simulink model "simulator"  (R2022b)
settings: Solver=FixedStepAuto  StartTime=0.0  StopTime=1800  FixedStep=1/7000  RelTol=1e-7
undefined symbols (not defined in the file): simdb
libraries: sim_lib x40, simulink_extras x15, matrix_library x9, simulink x1
(part 2 of 3)

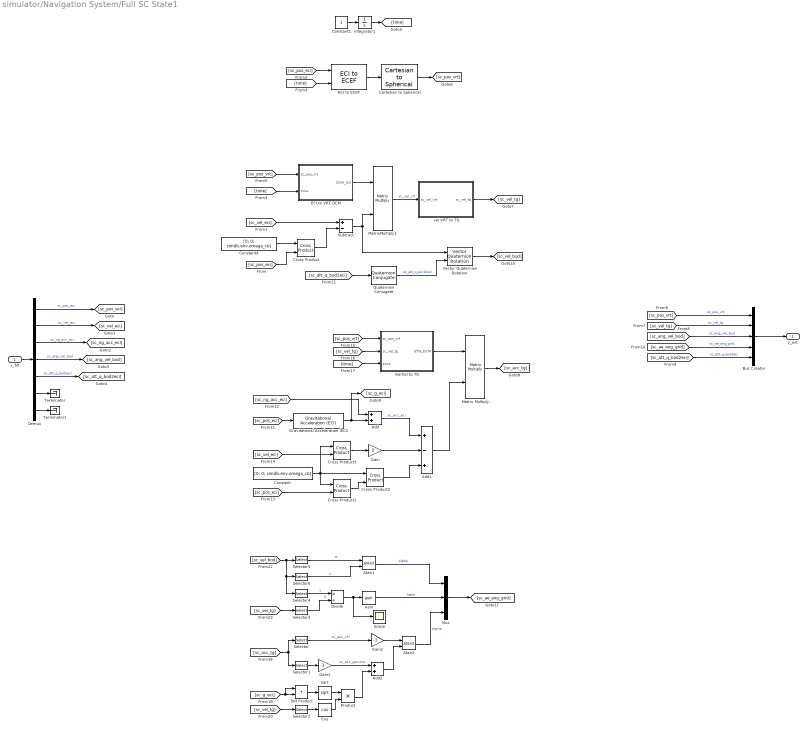
== system simulator/Navigation System/Full SC State1 ==
  x_filt : Inport
  Add : Sum
  Add1 : Sum  Inputs=+-+
  Add2 : Sum
  Asin : Trigonometry  Operator=asin
  Atan1 : Trigonometry  Operator=atan2
  Atan2 : Trigonometry  Operator=atan2
  Bus Creator : BusCreator  Inputs=5
  Cartesian to Spherical : sim_lib/Cartesian to Spherical  SystemSampleTime=-1  VariantActivationTime=update diagram  Latency=0  AutoFrameSizeCalculation=off
  Constant : Constant  Value=[0; 0; simdb.env.omega_cb]
  Constant1 : Constant
  Constant4 : Constant  Value=[0; 0; simdb.env.omega_cb]
  Cos : Trigonometry  Operator=cos
  Cross Product{,1..3} (4 alike) : matrix_library/Cross Product
  Demux : Demux  Outputs=7
  Divide : Product  Inputs=*/
  Dot Product : DotProduct  OutDataTypeStr=Inherit: Inherit via internal rule
  ECI to ECEF : sim_lib/ECI to ECEF  omega_cb=0
  ECI to VRT DCM : Subsystem
  Gain : Gain  Gain=2
  Gain1 : Gain  Gain=-1
  Gain2 : Gain  Gain=-1
  Gravitational Acceleration (ECI) : sim_lib/Gravitational Acceleration (ECI)  mu=simdb.env.mu
  Inertial to TG : Subsystem
  Integrator1 : Integrator
  Matrix Multiply : Product  Multiplication=Matrix(*)
  MatrixMultiply1 : Product  Multiplication=Matrix(*)
  Mux : Mux  Inputs=3
  Product : Product
  Quaternion Conjugate : sim_lib/Quaternion Conjugate  SystemSampleTime=-1  VariantActivationTime=update diagram  Latency=0  AutoFrameSizeCalculation=off
  Scope : Scope
  Selector : Selector  InputPortWidth=3  IndexOptions=Index vector (dialog)  Indices=[2]  OutputSizes=1
  Selector1 : Selector  InputPortWidth=3  IndexOptions=Index vector (dialog)  Indices=[3]  OutputSizes=1
  Selector2 : Selector  InputPortWidth=3  IndexOptions=Index vector (dialog)  Indices=[2]  OutputSizes=1
  Selector3 : Selector  InputPortWidth=3  IndexOptions=Index vector (dialog)  Indices=[1]  OutputSizes=1
  Selector4 : Selector  InputPortWidth=3  IndexOptions=Index vector (dialog)  Indices=[2]  OutputSizes=1
  Selector5 : Selector  InputPortWidth=3  IndexOptions=Index vector (dialog)  Indices=[3]  OutputSizes=1
  Selector6 : Selector  InputPortWidth=3  IndexOptions=Index vector (dialog)  Indices=[1]  OutputSizes=1
  Sqrt : Sqrt
  Subtract : Sum  Inputs=+-
  Terminator : Terminator
  Terminator1 : Terminator
  Vector Quaternion Rotation : sim_lib/Vector Quaternion Rotation  SystemSampleTime=-1  VariantActivationTime=update diagram  Latency=0  AutoFrameSizeCalculation=off
  vel VRT to TG : Subsystem
  y_est : Outport
  wires:
  x_filt/1 -> Demux/1
  Demux/2 -> [sc_vel_eci]  "sc_vel_eci"
  Demux/4 -> [sc_ang_vel_bod]  "sc_ang_vel_bod"
  Demux/5 -> [sc_att_q_bod2eci]  "sc_att_q_bod2eci"
  Demux/6 -> Terminator/1
  Demux/7 -> Terminator1/1
  Bus Creator/1 -> y_est/1
  Constant4/1 -> Cross Product/1
  Cross Product/1 -> Subtract/2
  Demux/1 -> [sc_pos_eci]  "sc_pos_eci"
  Demux/3 -> [sc_ng_acc_eci]  "sc_ng_acc_eci"
  [sc_pos_eci] -> Cross Product/2
  [sc_vel_eci] -> Subtract/1
  Subtract/1 -> MatrixMultiply1/2, Vector Quaternion Rotation/1
  ECI to VRT DCM/1(DCM_I2V) -> MatrixMultiply1/1
  Constant1/1 -> Integrator1/1
  Integrator1/1 -> [time]
  [time] -> ECI to VRT DCM/2(time)
  [sc_pos_eci] -> ECI to ECEF/1
  [time] -> ECI to ECEF/2
  ECI to ECEF/1 -> Cartesian to Spherical/1
  Cartesian to Spherical/1 -> [sc_pos_vrt]
  [sc_pos_vrt] -> ECI to VRT DCM/1(sc_pos_vrt)
  MatrixMultiply1/1 -> vel VRT to TG/1(sc_vel_vrt)  "sc_vel_vrt"
  vel VRT to TG/1(sc_vel_tg) -> [sc_vel_tg]
  [sc_pos_vrt] -> Bus Creator/1  "sc_pos_vrt"
  [sc_vel_tg] -> Bus Creator/2  "sc_vel_tg"
  [sc_ang_vel_bod] -> Bus Creator/3  "sc_ang_vel_bod"
  [sc_att_q_bod2eci] -> Bus Creator/5  "sc_att_q_bod2eci"
  [sc_ae_ang_gnd] -> Bus Creator/4  "sc_ae_ang_gnd"
  [sc_pos_eci] -> Gravitational Acceleration (ECI)/1
  Gravitational Acceleration (ECI)/1 -> Add/2, [sc_g_eci]
  [sc_ng_acc_eci] -> Add/1
  Add/1 -> Add1/1  "sc_acc_eci"
  [sc_pos_eci] -> Cross Product1/2
  Constant/1 -> Cross Product3/1, Cross Product2/1, Cross Product1/1
  Cross Product1/1 -> Cross Product2/2
  [sc_vel_eci] -> Cross Product3/2
  Cross Product3/1 -> Gain/1
  Gain/1 -> Add1/2
  Cross Product2/1 -> Add1/3
  Add1/1 -> Matrix Multiply/2
  [sc_pos_vrt] -> Inertial to TG/1(sc_pos_vrt)
  [sc_vel_tg] -> Inertial to TG/2(sc_vel_tg)
  [time] -> Inertial to TG/3(time)
  Inertial to TG/1(I2TG_DCM) -> Matrix Multiply/1
  Matrix Multiply/1 -> [sc_acc_tg]
  [sc_acc_tg] -> Selector/1, Selector1/1
  Selector/1 -> Gain2/1  "sc_acc_chi"
  Selector1/1 -> Gain1/1
  Gain1/1 -> Add2/1  "sc_acc_gamma"
  [sc_g_eci] -> Dot Product/1, Dot Product/2
  Dot Product/1 -> Sqrt/1
  [sc_vel_tg] -> Selector2/1
  Selector2/1 -> Cos/1
  Sqrt/1 -> Product/1
  Cos/1 -> Product/2
  Product/1 -> Add2/2
  Gain2/1 -> Atan2/1
  Add2/1 -> Atan2/2
  [sc_att_q_bod2eci] -> Quaternion Conjugate/1
  Quaternion Conjugate/1 -> Vector Quaternion Rotation/2  "sc_att_q_eci2bod"
  Vector Quaternion Rotation/1 -> [sc_vel_bod]
  [sc_vel_tg] -> Selector3/1
  [sc_vel_bod] -> Selector4/1, Selector6/1, Selector5/1
  Selector5/1 -> Atan1/1  "w"
  Selector6/1 -> Atan1/2  "u"
  Divide/1 -> Scope/1, Asin/1
  Selector4/1 -> Divide/1  "v"
  Selector3/1 -> Divide/2  "V"
  Atan1/1 -> Mux/1  "alpha"
  Asin/1 -> Mux/2  "beta"
  Atan2/1 -> Mux/3  "sigma"
  Mux/1 -> [sc_ae_ang_gnd]

== system simulator/Navigation System/IMU ==
  Bus Element In : Inport  PortName=dke_out  Element=sc_ng_acc_bod
  Bus Element In1 : Inport  PortName=dke_out  Element=sc_ang_vel_bod
  Accelerometer : Subsystem
  Gyroscope : Subsystem
  Terminator1 : Terminator
  Terminator2 : Terminator
  sen_acc_out : Outport
  sen_gyr_out : Outport  Port=2
  wires:
  Gyroscope/1(sen_gyr_out) -> sen_gyr_out/1
  Accelerometer/1(sen_acc_out) -> sen_acc_out/1
  Bus Element In/1 -> Accelerometer/1(sc_ng_acc_bod)
  Bus Element In1/1 -> Gyroscope/1(sc_ang_vel_bod)
  Gyroscope/2(sen_gyr_rawdata) -> Terminator2/1
  Accelerometer/2(sen_acc_rawdata) -> Terminator1/1

== system simulator/Plant/Aero-Surfaces Model ==
  delta_ae_cmd : Inport
  delta_ae : Outport
  wires:
  delta_ae_cmd/1 -> delta_ae/1

== system simulator/Plant/Forces & Moments ==
  state : Inport
  T : Inport  Port=2
  delta_ae : Inport  Port=3
  Aerodynamics : Subsystem
  Gravitational Force : Subsystem
  Height : sim_lib/Height  Rp=simdb.env.Rp
  RCS : Subsystem
  Selector : Selector  InputPortWidth=16  IndexOptions=Index vector (dialog)  Indices=[4]  OutputSizes=1
  Selector1 : Selector  InputPortWidth=16  IndexOptions=Index vector (dialog)  Indices=[1]  OutputSizes=1
  Selector2 : Selector  InputPortWidth=16  IndexOptions=Index vector (dialog)  Indices=[10]  OutputSizes=1
  Selector3 : Selector  InputPortWidth=16  IndexOptions=Index vector (dialog)  Indices=[11]  OutputSizes=1
  Selector4 : Selector  InputPortWidth=16  IndexOptions=Index vector (dialog)  Indices=[5]  OutputSizes=1
  Selector5 : Selector  InputPortWidth=16  IndexOptions=Index vector (dialog)  Indices=[12]  OutputSizes=1
  Bus Element Out : Outport  PortName=dyn_out  Element=sc_for_rcs_traj
  Bus Element Out1 : Outport  PortName=dyn_out  Element=sc_for_rcs_bod
  Bus Element Out2 : Outport  PortName=dyn_out  Element=sc_tor_rcs_bod
  Bus Element Out3 : Outport  PortName=dyn_out  Element=sc_for_g_traj
  Bus Element Out4 : Outport  PortName=dyn_out  Element=sc_for_ae_traj
  Bus Element Out5 : Outport  PortName=dyn_out  Element=sc_for_ae_bod
  Bus Element Out6 : Outport  PortName=dyn_out  Element=sc_tor_ae_bod
  wires:
  T/1 -> RCS/1(T)
  delta_ae/1 -> Aerodynamics/6(delta_ae)
  RCS/1(sc_for_rcs_traj) -> Bus Element Out/1
  RCS/3(sc_tor_rcs_bod) -> Bus Element Out2/1
  Gravitational Force/1(sc_for_g_traj) -> Bus Element Out3/1
  Selector1/1 -> Gravitational Force/1(R), Height/1  "R"
  Selector3/1 -> Aerodynamics/4(AoS)
  Selector/1 -> Aerodynamics/2(V)
  state/1 -> Selector5/1, Selector3/1, Selector2/1, Selector/1, Selector4/1, Selector1/1
  Selector4/1 -> Gravitational Force/2(gamma)
  Aerodynamics/3(sc_tor_ae_bod) -> Bus Element Out6/1
  Aerodynamics/1(sc_for_ae_traj) -> Bus Element Out4/1
  Height/1 -> Aerodynamics/1(h)
  RCS/2(sc_for_rcs_bod) -> Bus Element Out1/1
  Aerodynamics/2(sc_for_ae_bod) -> Bus Element Out5/1
  Selector2/1 -> Aerodynamics/3(AoA)
  Selector5/1 -> Aerodynamics/5(sigma)

== system simulator/Plant/Non-grav acceleration (bod) ==
  sc_pos_vrt : Inport
  sc_vel_tg : Inport  Port=2
  sc_att_q_bod2eci : Inport  Port=3
  dyn_out : Inport  Port=4
  Add : Sum
  Add1 : Sum
  Add2 : Sum
  Bus Selector2 : BusSelector  OutputSignals=sc_for_rcs_bod,sc_for_ae_bod
  Constant : Constant
  Cross Product : matrix_library/Cross Product
  Cross Product1 : matrix_library/Cross Product
  Cross Product2 : matrix_library/Cross Product
  Divide1 : Product  Inputs=*/
  ECEF to ECI : sim_lib/ECEF to ECI  omega_cb=0
  Gain : Gain  Gain=-1
  Gain1 : Gain  Gain=2
  Integrator : Integrator
  MatrixMultiply : Product  Multiplication=Matrix(*)
  Quaternion Conjugate : sim_lib/Quaternion Conjugate  SystemSampleTime=-1  VariantActivationTime=update diagram  Latency=0  AutoFrameSizeCalculation=off
  SPH 2 CART : sim_lib/Spherical to Cartesian  SystemSampleTime=-1  VariantActivationTime=update diagram  Latency=0  AutoFrameSizeCalculation=off
  VRT to ECI DCM : Subsystem
  Vector Quaternion Rotation : sim_lib/Vector Quaternion Rotation  SystemSampleTime=-1  VariantActivationTime=update diagram  Latency=0  AutoFrameSizeCalculation=off
  omega_cb_vec : Constant  Value=[0; 0; simdb.env.omega_cb]
  sc mass : Constant  Value=simdb.sc.m
  vel TG to VRT : Subsystem
  sc_ng_acc_bod : Outport
  wires:
  Constant/1 -> Integrator/1
  sc_pos_vrt/1 -> VRT to ECI DCM/1(sc_pos_vrt), SPH 2 CART/1
  sc_vel_tg/1 -> vel TG to VRT/1(sc_vel_tg)
  Integrator/1 -> ECEF to ECI/2, VRT to ECI DCM/2(time)
  VRT to ECI DCM/1(DCM_V2I) -> MatrixMultiply/1
  vel TG to VRT/1(sc_vel_vrt) -> MatrixMultiply/2
  MatrixMultiply/1 -> Cross Product2/2  "sc_vel_eci"
  SPH 2 CART/1 -> ECEF to ECI/1
  ECEF to ECI/1 -> Cross Product/2  "sc_pos_eci"
  omega_cb_vec/1 -> Cross Product1/1, Cross Product/1, Cross Product2/1
  Cross Product/1 -> Cross Product1/2
  Cross Product1/1 -> Gain/1
  Cross Product2/1 -> Gain1/1
  sc_att_q_bod2eci/1 -> Quaternion Conjugate/1
  Gain/1 -> Add1/1
  Gain1/1 -> Add1/2
  Add1/1 -> Vector Quaternion Rotation/1
  Quaternion Conjugate/1 -> Vector Quaternion Rotation/2
  dyn_out/1 -> Bus Selector2/1
  Bus Selector2/2 -> Add2/2  "<sc_for_ae_bod>"
  Add2/1 -> Divide1/1
  Bus Selector2/1 -> Add2/1  "<sc_for_rcs_bod>"
  sc mass/1 -> Divide1/2
  Vector Quaternion Rotation/1 -> Add/2
  Divide1/1 -> Add/1
  Add/1 -> sc_ng_acc_bod/1

== system simulator/Plant/Thrusters Model ==
  T_cmd : Inport
  T : Outport
  wires:
  T_cmd/1 -> T/1

== system simulator/Guidance System/Reference Trajectory/Ref Trajectory ==
  t : Inport
  Mux : Mux  Inputs=6
  Ref State (R) : Lookup_n-D  NumberOfTableDimensions=1  BreakpointsForDimension1=gui.t_gui  BreakpointsForDimension2=[1:3]  Table=gui.y_gui(1,:)  RemoveProtectionInput=on  InternalRulePriority=Speed  RndMeth=Simplest
  Ref State (V) : Lookup_n-D  NumberOfTableDimensions=1  BreakpointsForDimension1=gui.t_gui  BreakpointsForDimension2=[1:3]  Table=gui.y_gui(4,:)  RemoveProtectionInput=on  InternalRulePriority=Speed  RndMeth=Simplest
  Ref State (chi) : Lookup_n-D  NumberOfTableDimensions=1  BreakpointsForDimension1=gui.t_gui  BreakpointsForDimension2=[1:3]  Table=gui.y_gui(6,:)  RemoveProtectionInput=on  InternalRulePriority=Speed  RndMeth=Simplest
  Ref State (delta) : Lookup_n-D  NumberOfTableDimensions=1  BreakpointsForDimension1=gui.t_gui  BreakpointsForDimension2=[1:3]  Table=gui.y_gui(3,:)  RemoveProtectionInput=on  InternalRulePriority=Speed  RndMeth=Simplest
  Ref State (gamma) : Lookup_n-D  NumberOfTableDimensions=1  BreakpointsForDimension1=gui.t_gui  BreakpointsForDimension2=[1:3]  Table=gui.y_gui(5,:)  RemoveProtectionInput=on  InternalRulePriority=Speed  RndMeth=Simplest
  Ref State (tau) : Lookup_n-D  NumberOfTableDimensions=1  BreakpointsForDimension1=gui.t_gui  BreakpointsForDimension2=[1:3]  Table=gui.y_gui(2,:)  RemoveProtectionInput=on  InternalRulePriority=Speed  RndMeth=Simplest
  y_ref : Outport
  wires:
  t/1 -> Ref State (R)/1, Ref State (tau)/1, Ref State (delta)/1, Ref State (chi)/1, Ref State (gamma)/1, Ref State (V)/1
  Ref State (R)/1 -> Mux/1
  Ref State (chi)/1 -> Mux/6
  Ref State (tau)/1 -> Mux/2
  Ref State (delta)/1 -> Mux/3
  Ref State (V)/1 -> Mux/4
  Ref State (gamma)/1 -> Mux/5
  Mux/1 -> y_ref/1

== system simulator/Navigation System/Extended Kalman Filter/Covariance Matrix Estimation ==
  F : Inport
  P_prev : Inport  Port=2
  Add : Sum  Inputs=+++
  Matrix Multiply : Product  Multiplication=Matrix(*)
  Matrix Multiply1 : Product  Multiplication=Matrix(*)
  Q matrix : Constant  Value=simdb.nav.Q
  Transpose : Math  Operator=transpose
  P_est : Outport
  wires:
  F/1 -> Transpose/1, Matrix Multiply/1
  Matrix Multiply1/1 -> Add/1
  Matrix Multiply/1 -> Add/2
  P_prev/1 -> Matrix Multiply/2, Matrix Multiply1/1
  Q matrix/1 -> Add/3
  Add/1 -> P_est/1
  Transpose/1 -> Matrix Multiply1/2

== system simulator/Navigation System/Extended Kalman Filter/Covariance Matrix Update ==
  K : Inport
  H : Inport  Port=2
  P_est : Inport  Port=3
  Identity : Constant  Value=eye(22)
  Matrix Multiply : Product  Multiplication=Matrix(*)
  Matrix Multiply1 : Product  Multiplication=Matrix(*)
  Subtract : Sum  Inputs=+-
  P_new : Outport
  wires:
  H/1 -> Matrix Multiply/2
  K/1 -> Matrix Multiply/1
  Identity/1 -> Subtract/1
  Matrix Multiply/1 -> Subtract/2
  Subtract/1 -> Matrix Multiply1/1
  P_est/1 -> Matrix Multiply1/2
  Matrix Multiply1/1 -> P_new/1

== system simulator/Navigation System/Extended Kalman Filter/Kalman Gain ==
  H : Inport
  P_est : Inport  Port=2
  Add1 : Sum
  Matrix Multiply2 : Product  Multiplication=Matrix(*)
  Matrix Multiply3 : Product  Multiplication=Matrix(*)
  Matrix Multiply4 : Product  Multiplication=Matrix(*)
  Product : Product  Inputs=*/  Multiplication=Matrix(*)
  R Matrix : Constant  Value=simdb.nav.R
  Transpose1 : Math  Operator=transpose
  K : Outport
  wires:
  H/1 -> Transpose1/1, Matrix Multiply2/1
  Matrix Multiply3/1 -> Add1/2
  Matrix Multiply2/1 -> Matrix Multiply3/1
  Transpose1/1 -> Product/1, Matrix Multiply3/2
  R Matrix/1 -> Add1/1
  Product/1 -> Matrix Multiply4/2
  P_est/1 -> Matrix Multiply4/1, Matrix Multiply2/2
  Add1/1 -> Product/2
  Matrix Multiply4/1 -> K/1

== system simulator/Navigation System/Full SC State/ECI to VRT DCM ==
  sc_pos_vrt : Inport
  time : Inport  Port=2
  Add : Sum
  Add1 : Sum
  C2_delta : sim_lib/Ry DCM  SystemSampleTime=-1  VariantActivationTime=update diagram  Latency=0  AutoFrameSizeCalculation=off
  C3_tau : sim_lib/Rz DCM  SystemSampleTime=-1  VariantActivationTime=update diagram  Latency=0  AutoFrameSizeCalculation=off
  Constant : Constant  Value=pi/2
  Gain1 : Gain  Gain=-1
  MatrixMultiply : Product  Multiplication=Matrix(*)
  delta : Selector  InputPortWidth=3  IndexOptions=Index vector (dialog)  Indices=[3]  OutputSizes=1
  omega_cb : Gain  Gain=simdb.env.omega_cb
  tau : Selector  InputPortWidth=3  IndexOptions=Index vector (dialog)  Indices=[2]  OutputSizes=1
  DCM_I2V : Outport
  wires:
  sc_pos_vrt/1 -> delta/1, tau/1
  time/1 -> omega_cb/1
  tau/1 -> Add/1
  omega_cb/1 -> Add/2
  delta/1 -> Add1/2
  Constant/1 -> Add1/1
  Add1/1 -> Gain1/1
  Gain1/1 -> C2_delta/1
  Add/1 -> C3_tau/1
  C3_tau/1 -> MatrixMultiply/2
  C2_delta/1 -> MatrixMultiply/1
  MatrixMultiply/1 -> DCM_I2V/1

== system simulator/Navigation System/Full SC State/Inertial to TG ==
  sc_pos_vrt : Inport
  sc_vel_tg : Inport  Port=2
  time : Inport  Port=3
  Add : Sum
  Add1 : Sum
  C2_delta : sim_lib/Ry DCM  SystemSampleTime=-1  VariantActivationTime=update diagram  Latency=0  AutoFrameSizeCalculation=off
  C2_gamma : sim_lib/Ry DCM  SystemSampleTime=-1  VariantActivationTime=update diagram  Latency=0  AutoFrameSizeCalculation=off
  C3_chi : sim_lib/Rz DCM  SystemSampleTime=-1  VariantActivationTime=update diagram  Latency=0  AutoFrameSizeCalculation=off
  C3_tau_omega : sim_lib/Rz DCM  SystemSampleTime=-1  VariantActivationTime=update diagram  Latency=0  AutoFrameSizeCalculation=off
  Constant : Constant  Value=pi/2
  Gain : Gain  Gain=-1
  Matrix Multiply : Product  Multiplication=Matrix(*)
  Matrix Multiply1 : Product  Multiplication=Matrix(*)
  Matrix Multiply2 : Product  Multiplication=Matrix(*)
  Selector : Selector  InputPortWidth=3  IndexOptions=Index vector (dialog)  Indices=[2]  OutputSizes=1
  Selector1 : Selector  InputPortWidth=3  IndexOptions=Index vector (dialog)  Indices=[3]  OutputSizes=1
  Selector2 : Selector  InputPortWidth=3  IndexOptions=Index vector (dialog)  Indices=[2]  OutputSizes=1
  Selector3 : Selector  InputPortWidth=3  IndexOptions=Index vector (dialog)  Indices=[3]  OutputSizes=1
  I2TG_DCM : Outport
  wires:
  sc_pos_vrt/1 -> Selector/1, Selector1/1
  Selector1/1 -> Add1/2  "delta"
  sc_vel_tg/1 -> Selector2/1, Selector3/1
  time/1 -> Add/2
  Selector/1 -> Add/1  "tau"
  Constant/1 -> Add1/1
  Add1/1 -> Gain/1
  Add/1 -> C3_tau_omega/1
  Gain/1 -> C2_delta/1
  C3_tau_omega/1 -> Matrix Multiply/2
  C2_delta/1 -> Matrix Multiply/1
  Selector3/1 -> C3_chi/1  "chi"
  Matrix Multiply/1 -> Matrix Multiply1/2
  C3_chi/1 -> Matrix Multiply1/1
  Selector2/1 -> C2_gamma/1  "gamma"
  Matrix Multiply1/1 -> Matrix Multiply2/2
  C2_gamma/1 -> Matrix Multiply2/1
  Matrix Multiply2/1 -> I2TG_DCM/1

== system simulator/Navigation System/Full SC State/Rotation Vector (Vertical Frame) ==
  sc_pos_vrt : Inport
  time : Inport  Port=2
  Add : Sum
  Add1 : Sum
  Divide : Product  Inputs=/*
  Divide1 : Product  Inputs=/*
  Gain : Gain  Gain=-1
  Memory : Memory  InitialCondition=simdb.nav.sc_pos_vrt_init(2)
  Memory1 : Memory  InitialCondition=simdb.nav.sc_pos_vrt_init(3)
  Memory2 : Memory  InitialCondition=1/7000
  Mux : Mux  Inputs=3
  Product : Product
  Product1 : Product
  Product2 : Product
  SinCos : Trigonometry  Operator=sincos
  Sum : Sum  Inputs=|+-
  Sum1 : Sum  Inputs=|+-
  Sum2 : Sum  Inputs=|+-
  delta : Selector  InputPortWidth=3  IndexOptions=Index vector (dialog)  Indices=[3]  OutputSizes=1
  omega_cb : Constant  Value=simdb.env.omega_cb
  tau : Selector  InputPortWidth=3  IndexOptions=Index vector (dialog)  Indices=[2]  OutputSizes=1
  rot_vec_vrt : Outport
  wires:
  sc_pos_vrt/1 -> tau/1, delta/1
  delta/1 -> Sum1/1, Memory1/1
  tau/1 -> Add/2, Memory/1, Sum/1
  Add/1 -> SinCos/1
  Product/1 -> Add/1
  Product2/1 -> Gain/1
  SinCos/2 -> Product2/2
  omega_cb/1 -> Product/2
  Mux/1 -> rot_vec_vrt/1
  Memory/1 -> Sum/2
  Add1/1 -> Mux/3
  Sum1/1 -> Divide/2, Product2/1  "delta_dot"
  SinCos/1 -> Product1/2
  Memory1/1 -> Sum1/2
  Memory2/1 -> Sum2/2
  time/1 -> Memory2/1, Sum2/1, Product/1
  Divide/1 -> Product1/1
  Sum2/1 -> Divide/1, Divide1/1  "dt"
  Sum/1 -> Divide1/2  "tau_dot"
  Divide1/1 -> Add1/2
  Product1/1 -> Mux/1
  Gain/1 -> Mux/2

== system simulator/Navigation System/Full SC State/Subsystem ==
  C_B2TG : Inport
  Asin : Trigonometry  Operator=asin
  Atan1 : Trigonometry  Operator=atan2
  Atan2 : Trigonometry  Operator=atan2
  Demux : Demux  Outputs=9
  Gain : Gain  Gain=-1
  Mux : Mux  Inputs=3
  Reshape : Reshape
  Terminator{,1..3} (4 alike) : Terminator
  sc_ae_ang_gnd : Outport
  wires:
  C_B2TG/1 -> Reshape/1
  Reshape/1 -> Demux/1
  Mux/1 -> sc_ae_ang_gnd/1
  Demux/6 -> Gain/1
  Demux/5 -> Atan2/2
  Gain/1 -> Atan2/1
  Atan2/1 -> Mux/3
  Atan1/1 -> Mux/1
  Demux/7 -> Atan1/1
  Demux/1 -> Atan1/2
  Asin/1 -> Mux/2
  Demux/4 -> Asin/1
  Demux/2 -> Terminator/1
  Demux/3 -> Terminator1/1
  Demux/8 -> Terminator2/1
  Demux/9 -> Terminator3/1

== system simulator/Navigation System/Full SC State/vel VRT to TG ==
  sc_vel_vrt : Inport
  Asin : Trigonometry  Operator=asin
  Atan2 : Trigonometry  Operator=atan2
  Demux : Demux  Outputs=3
  Divide : Product  Inputs=/*
  Dot Product : DotProduct  OutDataTypeStr=Inherit: Inherit via internal rule
  Gain : Gain  Gain=-1
  Mux : Mux  Inputs=3
  Sqrt : Sqrt
  sc_vel_tg : Outport
  wires:
  Sqrt/1 -> Divide/1, Mux/1
  Dot Product/1 -> Sqrt/1
  Mux/1 -> sc_vel_tg/1
  sc_vel_vrt/1 -> Demux/1, Dot Product/1, Dot Product/2
  Demux/2 -> Atan2/1
  Divide/1 -> Gain/1
  Demux/1 -> Atan2/2
  Atan2/1 -> Mux/3
  Asin/1 -> Mux/2
  Demux/3 -> Divide/2
  Gain/1 -> Asin/1

== system simulator/Navigation System/Full SC State1/ECI to VRT DCM ==
  sc_pos_vrt : Inport
  time : Inport  Port=2
  Add : Sum
  Add1 : Sum
  C2_delta : sim_lib/Ry DCM  SystemSampleTime=-1  VariantActivationTime=update diagram  Latency=0  AutoFrameSizeCalculation=off
  C3_tau : sim_lib/Rz DCM  SystemSampleTime=-1  VariantActivationTime=update diagram  Latency=0  AutoFrameSizeCalculation=off
  Constant : Constant  Value=pi/2
  Gain1 : Gain  Gain=-1
  MatrixMultiply : Product  Multiplication=Matrix(*)
  delta : Selector  InputPortWidth=3  IndexOptions=Index vector (dialog)  Indices=[3]  OutputSizes=1
  omega_cb : Gain  Gain=simdb.env.omega_cb
  tau : Selector  InputPortWidth=3  IndexOptions=Index vector (dialog)  Indices=[2]  OutputSizes=1
  DCM_I2V : Outport
  wires:
  sc_pos_vrt/1 -> delta/1, tau/1
  time/1 -> omega_cb/1
  tau/1 -> Add/1
  omega_cb/1 -> Add/2
  delta/1 -> Add1/2
  Constant/1 -> Add1/1
  Add1/1 -> Gain1/1
  Gain1/1 -> C2_delta/1
  Add/1 -> C3_tau/1
  C3_tau/1 -> MatrixMultiply/2
  C2_delta/1 -> MatrixMultiply/1
  MatrixMultiply/1 -> DCM_I2V/1

== system simulator/Navigation System/Full SC State1/Inertial to TG ==
  sc_pos_vrt : Inport
  sc_vel_tg : Inport  Port=2
  time : Inport  Port=3
  Add : Sum
  Add1 : Sum
  C2_delta : sim_lib/Ry DCM  SystemSampleTime=-1  VariantActivationTime=update diagram  Latency=0  AutoFrameSizeCalculation=off
  C2_gamma : sim_lib/Ry DCM  SystemSampleTime=-1  VariantActivationTime=update diagram  Latency=0  AutoFrameSizeCalculation=off
  C3_chi : sim_lib/Rz DCM  SystemSampleTime=-1  VariantActivationTime=update diagram  Latency=0  AutoFrameSizeCalculation=off
  C3_tau_omega : sim_lib/Rz DCM  SystemSampleTime=-1  VariantActivationTime=update diagram  Latency=0  AutoFrameSizeCalculation=off
  Constant : Constant  Value=pi/2
  Gain : Gain  Gain=-1
  Matrix Multiply : Product  Multiplication=Matrix(*)
  Matrix Multiply1 : Product  Multiplication=Matrix(*)
  Matrix Multiply2 : Product  Multiplication=Matrix(*)
  Selector : Selector  InputPortWidth=3  IndexOptions=Index vector (dialog)  Indices=[2]  OutputSizes=1
  Selector1 : Selector  InputPortWidth=3  IndexOptions=Index vector (dialog)  Indices=[3]  OutputSizes=1
  Selector2 : Selector  InputPortWidth=3  IndexOptions=Index vector (dialog)  Indices=[2]  OutputSizes=1
  Selector3 : Selector  InputPortWidth=3  IndexOptions=Index vector (dialog)  Indices=[3]  OutputSizes=1
  I2TG_DCM : Outport
  wires:
  sc_pos_vrt/1 -> Selector/1, Selector1/1
  Selector1/1 -> Add1/2  "delta"
  sc_vel_tg/1 -> Selector2/1, Selector3/1
  time/1 -> Add/2
  Selector/1 -> Add/1  "tau"
  Constant/1 -> Add1/1
  Add1/1 -> Gain/1
  Add/1 -> C3_tau_omega/1
  Gain/1 -> C2_delta/1
  C3_tau_omega/1 -> Matrix Multiply/2
  C2_delta/1 -> Matrix Multiply/1
  Selector3/1 -> C3_chi/1  "chi"
  Matrix Multiply/1 -> Matrix Multiply1/2
  C3_chi/1 -> Matrix Multiply1/1
  Selector2/1 -> C2_gamma/1  "gamma"
  Matrix Multiply1/1 -> Matrix Multiply2/2
  C2_gamma/1 -> Matrix Multiply2/1
  Matrix Multiply2/1 -> I2TG_DCM/1

== system simulator/Navigation System/Full SC State1/vel VRT to TG ==
  sc_vel_vrt : Inport
  Asin : Trigonometry  Operator=asin
  Atan2 : Trigonometry  Operator=atan2
  Demux : Demux  Outputs=3
  Divide : Product  Inputs=/*
  Dot Product : DotProduct  OutDataTypeStr=Inherit: Inherit via internal rule
  Gain : Gain  Gain=-1
  Mux : Mux  Inputs=3
  Sqrt : Sqrt
  sc_vel_tg : Outport
  wires:
  Sqrt/1 -> Divide/1, Mux/1
  Dot Product/1 -> Sqrt/1
  Mux/1 -> sc_vel_tg/1
  sc_vel_vrt/1 -> Demux/1, Dot Product/1, Dot Product/2
  Demux/2 -> Atan2/1
  Divide/1 -> Gain/1
  Demux/1 -> Atan2/2
  Atan2/1 -> Mux/3
  Asin/1 -> Mux/2
  Demux/3 -> Divide/2
  Gain/1 -> Asin/1

== system simulator/Navigation System/IMU/Accelerometer ==
  sc_ng_acc_bod : Inport
  ADC Quantization Error : Quantizer  QuantizationInterval=acc.quant_res
  Acc Saturation : Saturate  UpperLimit=acc.max_acc  LowerLimit=-acc.max_acc
  Bus Creator : BusCreator  Inputs=2
  Bus Creator1 : BusCreator  Inputs=2
  Internal Sampling : ZeroOrderHold  SampleTime=acc.internal_tsample
  Latency : TransportDelay  DelayTime=gyr.output_delay
  Latency1 : TransportDelay  DelayTime=gyr.output_delay
  Rate Transition1 : RateTransition  OutPortSampleTime=acc.output_tsample
  Velocity Increment : Subsystem
  sen_acc_out : Outport
  sen_acc_rawdata : Outport  Port=2
  wires:
  Bus Creator/1 -> sen_acc_out/1
  sc_ng_acc_bod/1 -> [sc_ng_acc_bod_ideal], ADC Quantization Error/1
  Bus Creator1/1 -> sen_acc_rawdata/1
  Latency/1 -> Bus Creator/2  "sc_inc_ng_vel_bod"
  Latency1/1 -> [sc_ng_acc_bod_meas], Bus Creator/1  "sc_ng_acc_bod"
  Velocity Increment/1(sc_inc_ng_vel_bod) -> Latency/1
  Rate Transition1/1 -> Latency1/1
  Acc Saturation/1 -> Internal Sampling/1
  ADC Quantization Error/1 -> Acc Saturation/1
  Internal Sampling/1 -> Rate Transition1/1, Velocity Increment/1(sc_ng_acc_bod)
  [sc_ng_acc_bod_ideal] -> Bus Creator1/1  "sc_ng_acc_bod_ideal"
  [sc_ng_acc_bod_meas] -> Bus Creator1/2  "sc_ng_acc_bod_meas"

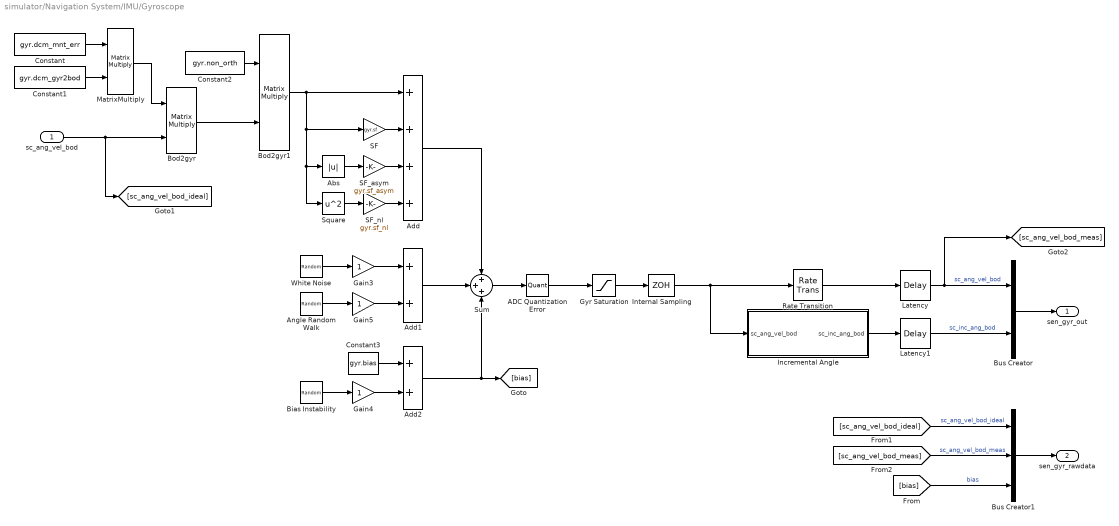
== system simulator/Navigation System/IMU/Gyroscope ==
  sc_ang_vel_bod : Inport
  ADC Quantization Error : Quantizer  QuantizationInterval=gyr.quant_res
  Abs : Abs  SaturateOnIntegerOverflow=off
  Add : Sum  Inputs=++++
  Add1 : Sum
  Add2 : Sum
  Angle Random Walk : RandomNumber  Mean=gyr.ARW_mu  Variance=gyr.ARW_var  Seed=gyr.ARW_seed  SampleTime=0
  Bias Instability : RandomNumber  Mean=gyr.bias_inst_mu  Variance=gyr.bias_inst_var  Seed=gyr.bias_inst_seed  SampleTime=0
  Bod2gyr : Product  Multiplication=Matrix(*)
  Bod2gyr1 : Product  Multiplication=Matrix(*)
  Bus Creator : BusCreator  Inputs=2
  Bus Creator1 : BusCreator  Inputs=3
  Constant : Constant  Value=gyr.dcm_mnt_err
  Constant1 : Constant  Value=gyr.dcm_gyr2bod
  Constant2 : Constant  Value=gyr.non_orth
  Constant3 : Constant  Value=gyr.bias
  Gain3 : Gain
  Gain4 : Gain
  Gain5 : Gain
  Gyr Saturation : Saturate  UpperLimit=gyr.max_ang_vel  LowerLimit=-gyr.max_ang_vel
  Incremental Angle : Subsystem
  Internal Sampling : ZeroOrderHold  SampleTime=gyr.internal_tsample
  Latency : TransportDelay  DelayTime=gyr.output_delay
  Latency1 : TransportDelay  DelayTime=gyr.output_delay
  MatrixMultiply : Product  Multiplication=Matrix(*)
  Rate Transition : RateTransition  OutPortSampleTime=gyr.output_tsample
  SF : Gain  Gain=gyr.sf
  SF_asym : Gain  Gain=gyr.sf_asym
  SF_nl : Gain  Gain=gyr.sf_nl
  Square : Math  Operator=square
  Sum : Sum  Inputs=+++
  White Noise : RandomNumber  Mean=gyr.white_noise_mu  Variance=gyr.white_noise_var  Seed=gyr.white_noise_seed  SampleTime=0
  sen_gyr_out : Outport
  sen_gyr_rawdata : Outport  Port=2
  wires:
  Constant/1 -> MatrixMultiply/1
  Constant1/1 -> MatrixMultiply/2
  sc_ang_vel_bod/1 -> [sc_ang_vel_bod_ideal], Bod2gyr/2
  MatrixMultiply/1 -> Bod2gyr/1
  Bod2gyr/1 -> Bod2gyr1/2
  Constant2/1 -> Bod2gyr1/1
  Bod2gyr1/1 -> Square/1, Abs/1, SF/1, Add/1
  SF/1 -> Add/2
  Square/1 -> SF_nl/1
  SF_nl/1 -> Add/4
  SF_asym/1 -> Add/3
  Abs/1 -> SF_asym/1
  White Noise/1 -> Gain3/1
  Bias Instability/1 -> Gain4/1
  Gain3/1 -> Add1/1
  Gain5/1 -> Add1/2
  Angle Random Walk/1 -> Gain5/1
  Sum/1 -> ADC Quantization Error/1
  ADC Quantization Error/1 -> Gyr Saturation/1
  Gyr Saturation/1 -> Internal Sampling/1
  Bus Creator/1 -> sen_gyr_out/1
  Internal Sampling/1 -> Incremental Angle/1(sc_ang_vel_bod), Rate Transition/1
  Constant3/1 -> Add2/1
  Gain4/1 -> Add2/2
  Add/1 -> Sum/1
  Add1/1 -> Sum/2
  Add2/1 -> [bias], Sum/3
  Latency/1 -> [sc_ang_vel_bod_meas], Bus Creator/1  "sc_ang_vel_bod"
  Latency1/1 -> Bus Creator/2  "sc_inc_ang_bod"
  Incremental Angle/1(sc_inc_ang_bod) -> Latency1/1
  Rate Transition/1 -> Latency/1
  Bus Creator1/1 -> sen_gyr_rawdata/1
  [bias] -> Bus Creator1/3  "bias"
  [sc_ang_vel_bod_ideal] -> Bus Creator1/1  "sc_ang_vel_bod_ideal"
  [sc_ang_vel_bod_meas] -> Bus Creator1/2  "sc_ang_vel_bod_meas"

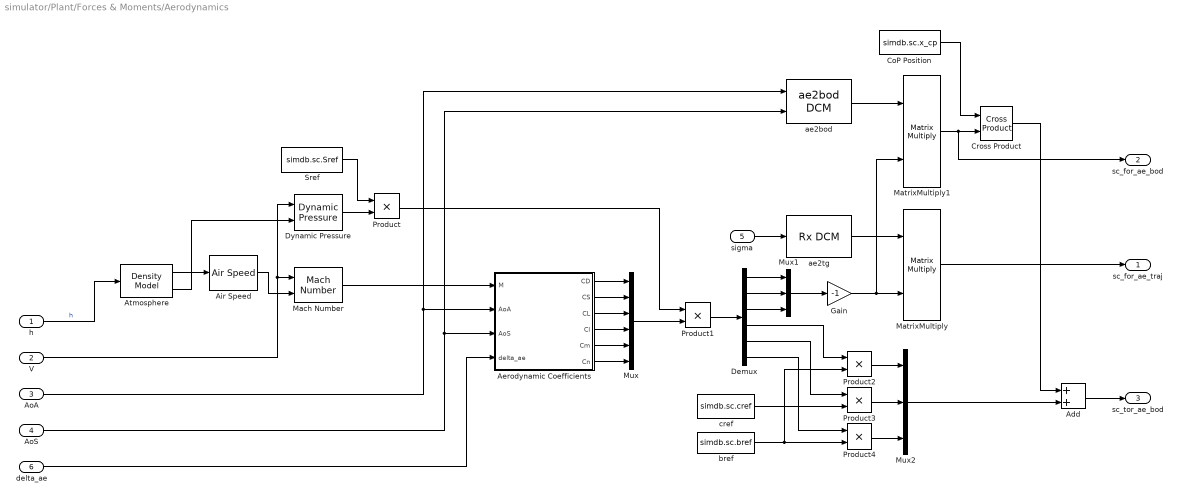
== system simulator/Plant/Forces & Moments/Aerodynamics ==
  h : Inport
  V : Inport  Port=2
  AoA : Inport  Port=3
  AoS : Inport  Port=4
  sigma : Inport  Port=5
  delta_ae : Inport  Port=6
  Add : Sum
  Aerodynamic Coefficients : Subsystem
  Air Speed : sim_lib/Air Speed  Rg=simdb.env.Rg  gamma=simdb.env.gamma
  Atmosphere : sim_lib/Density Model  h_base=simdb.env.h_base  T_base=simdb.env.T_base  rho_base=simdb.env.rho_base
  CoP Position : Constant  Value=simdb.sc.x_cp
  Cross Product : matrix_library/Cross Product
  Demux : Demux  Outputs=6
  Dynamic Pressure : sim_lib/Dynamic Pressure  SystemSampleTime=-1  VariantActivationTime=update diagram  Latency=0  AutoFrameSizeCalculation=off
  Gain : Gain  Gain=-1
  Mach Number : sim_lib/Mach Number  SystemSampleTime=-1  VariantActivationTime=update diagram  Latency=0  AutoFrameSizeCalculation=off
  MatrixMultiply : Product  Multiplication=Matrix(*)
  MatrixMultiply1 : Product  Multiplication=Matrix(*)
  Mux : Mux  Inputs=6
  Mux1 : Mux  Inputs=3
  Mux2 : Mux  Inputs=3
  Product{,1..4} (5 alike) : Product
  Sref : Constant  Value=simdb.sc.Sref
  ae2bod : sim_lib/ae2bod DCM  SystemSampleTime=-1  VariantActivationTime=update diagram  Latency=0  AutoFrameSizeCalculation=off
  ae2tg : sim_lib/Rx DCM  SystemSampleTime=-1  VariantActivationTime=update diagram  Latency=0  AutoFrameSizeCalculation=off
  bref : Constant  Value=simdb.sc.bref
  cref : Constant  Value=simdb.sc.cref
  sc_for_ae_traj : Outport
  sc_for_ae_bod : Outport  Port=2
  sc_tor_ae_bod : Outport  Port=3
  wires:
  Atmosphere/1 -> Air Speed/1
  h/1 -> Atmosphere/1  "h"
  Air Speed/1 -> Mach Number/2
  V/1 -> Mach Number/1, Dynamic Pressure/1
  Atmosphere/2 -> Dynamic Pressure/2
  Mach Number/1 -> Aerodynamic Coefficients/1(M)
  AoA/1 -> ae2bod/1, Aerodynamic Coefficients/2(AoA)
  AoS/1 -> ae2bod/2, Aerodynamic Coefficients/3(AoS)
  delta_ae/1 -> Aerodynamic Coefficients/4(delta_ae)
  Dynamic Pressure/1 -> Product/2
  Sref/1 -> Product/1
  Aerodynamic Coefficients/5(Cm) -> Mux/5
  Aerodynamic Coefficients/6(Cn) -> Mux/6
  Aerodynamic Coefficients/4(Cl) -> Mux/4
  Aerodynamic Coefficients/3(CL) -> Mux/3
  Aerodynamic Coefficients/2(CS) -> Mux/2
  Aerodynamic Coefficients/1(CD) -> Mux/1
  Mux/1 -> Product1/2
  Product/1 -> Product1/1
  Product1/1 -> Demux/1
  Demux/1 -> Mux1/1
  Demux/2 -> Mux1/2
  Demux/3 -> Mux1/3
  Demux/5 -> Product3/1
  Demux/6 -> Product4/1
  Demux/4 -> Product2/1
  cref/1 -> Product3/2
  bref/1 -> Product2/2, Product4/2
  Product2/1 -> Mux2/1
  Product3/1 -> Mux2/2
  Product4/1 -> Mux2/3
  Mux2/1 -> Add/2
  sigma/1 -> ae2tg/1
  Mux1/1 -> Gain/1
  Gain/1 -> MatrixMultiply/2, MatrixMultiply1/2
  ae2bod/1 -> MatrixMultiply1/1
  MatrixMultiply1/1 -> sc_for_ae_bod/1, Cross Product/2
  CoP Position/1 -> Cross Product/1
  Add/1 -> sc_tor_ae_bod/1
  Cross Product/1 -> Add/1
  MatrixMultiply/1 -> sc_for_ae_traj/1
  ae2tg/1 -> MatrixMultiply/1

== system simulator/Plant/Forces & Moments/Gravitational Force ==
  R : Inport
  gamma : Inport  Port=2
  Constant : Constant  Value=0
  Gain : Gain  Gain=simdb.sc.m
  Gain2 : Gain  Gain=-1
  Mux : Mux  Inputs=3
  Product : Product  Inputs=*/
  Product1 : Product
  Product2 : Product
  SinCos : Trigonometry  Operator=sincos
  Square : Math  Operator=square
  mu : Constant  Value=simdb.env.mu
  sc_for_g_traj : Outport
  wires:
  Square/1 -> Product/2
  R/1 -> Square/1
  mu/1 -> Product/1
  Product/1 -> Gain/1
  Product1/1 -> Gain2/1
  Product2/1 -> Mux/3
  Constant/1 -> Mux/2
  Gain2/1 -> Mux/1
  Gain/1 -> Product2/2, Product1/2
  SinCos/1 -> Product1/1
  SinCos/2 -> Product2/1
  Mux/1 -> sc_for_g_traj/1
  gamma/1 -> SinCos/1

== system simulator/Plant/Forces & Moments/RCS ==
  T : Inport
  Constant : Constant  Value=[0; 0; 0]
  sc_for_rcs_traj : Outport
  sc_for_rcs_bod : Outport  Port=2
  sc_tor_rcs_bod : Outport  Port=3
  wires:
  T/1 -> sc_tor_rcs_bod/1
  Constant/1 -> sc_for_rcs_bod/1, sc_for_rcs_traj/1

== system simulator/Plant/Non-grav acceleration (bod)/VRT to ECI DCM ==
  sc_pos_vrt : Inport
  time : Inport  Port=2
  Add : Sum
  Add1 : Sum
  C2_delta : sim_lib/Ry DCM  SystemSampleTime=-1  VariantActivationTime=update diagram  Latency=0  AutoFrameSizeCalculation=off
  C3_tau : sim_lib/Rz DCM  SystemSampleTime=-1  VariantActivationTime=update diagram  Latency=0  AutoFrameSizeCalculation=off
  Constant : Constant  Value=pi/2
  Gain1 : Gain  Gain=-1
  MatrixMultiply : Product  Multiplication=Matrix(*)
  delta : Selector  InputPortWidth=3  IndexOptions=Index vector (dialog)  Indices=[3]  OutputSizes=1
  omega_cb : Gain  Gain=simdb.env.omega_cb
  tau : Selector  InputPortWidth=3  IndexOptions=Index vector (dialog)  Indices=[2]  OutputSizes=1
  DCM_V2I : Outport
  wires:
  sc_pos_vrt/1 -> tau/1, delta/1
  time/1 -> omega_cb/1
  Add/1 -> Gain1/1
  MatrixMultiply/1 -> DCM_V2I/1
  tau/1 -> Add/2
  omega_cb/1 -> Add/1
  Gain1/1 -> C3_tau/1
  Add1/1 -> C2_delta/1
  delta/1 -> Add1/1
  Constant/1 -> Add1/2
  C2_delta/1 -> MatrixMultiply/2
  C3_tau/1 -> MatrixMultiply/1

== system simulator/Plant/Non-grav acceleration (bod)/vel TG to VRT ==
  sc_vel_tg : Inport
  Demux : Demux  Outputs=3
  Gain : Gain  Gain=-1
  Mux : Mux  Inputs=3
  Product : Product  Inputs=3
  Product1 : Product  Inputs=3
  Product2 : Product
  SinCos : Trigonometry  Operator=sincos
  SinCos1 : Trigonometry  Operator=sincos
  sc_vel_vrt : Outport
  wires:
  sc_vel_tg/1 -> Demux/1
  Demux/2 -> SinCos/1  "gamma"
  Demux/3 -> SinCos1/1  "chi"
  Mux/1 -> sc_vel_vrt/1
  Product/1 -> Mux/1
  Product1/1 -> Mux/2
  Product2/1 -> Gain/1
  Demux/1 -> Product2/1, Product1/1, Product/1  "V"
  Gain/1 -> Mux/3
  SinCos/2 -> Product1/3, Product/3
  SinCos/1 -> Product2/2
  SinCos1/1 -> Product1/2
  SinCos1/2 -> Product/2

== system simulator/Navigation System/IMU/Accelerometer/Velocity Increment ==
  sc_ng_acc_bod : Inport
  Constant : Constant  Value=2
  Delay One Step : Delay  DelayLength=1
  Merge : Merge
  Perfect Integration : Subsystem  TreatAsAtomicUnit=on
  Rate Transition : RateTransition  OutPortSampleTime=acc.output_tsample
  Sum : Sum  Inputs=|+-
  Switch Case : SwitchCase  CaseConditions={1,2}  ShowDefaultCase=off
  Trapezoid Integration : Subsystem  TreatAsAtomicUnit=on
  sc_inc_ng_vel_bod : Outport
  wires:
  Constant/1 -> Switch Case/1
  Switch Case/1 -> Trapezoid Integration/Action
  Delay One Step/1 -> Sum/2
  Trapezoid Integration/1(out) -> Merge/1
  Perfect Integration/1(out) -> Merge/2
  Sum/1 -> sc_inc_ng_vel_bod/1
  Switch Case/2 -> Perfect Integration/Action
  Rate Transition/1 -> Sum/1, Delay One Step/1
  Merge/1 -> Rate Transition/1
  sc_ng_acc_bod/1 -> Perfect Integration/1(in), Trapezoid Integration/1(in)

== system simulator/Navigation System/IMU/Gyroscope/Incremental Angle ==
  sc_ang_vel_bod : Inport
  Constant : Constant  Value=2
  Delay One Step : Delay  DelayLength=1
  Merge : Merge
  Perfect Integration : Subsystem  TreatAsAtomicUnit=on
  Rate Transition : RateTransition  OutPortSampleTime=gyr.output_tsample
  Sum : Sum  Inputs=|+-
  Switch Case : SwitchCase  CaseConditions={1,2}  ShowDefaultCase=off
  Trapezoid Integration : Subsystem  TreatAsAtomicUnit=on
  sc_inc_ang_bod : Outport
  wires:
  Constant/1 -> Switch Case/1
  Switch Case/1 -> Trapezoid Integration/Action
  Switch Case/2 -> Perfect Integration/Action
  Perfect Integration/1(out) -> Merge/2
  Trapezoid Integration/1(out) -> Merge/1
  sc_ang_vel_bod/1 -> Perfect Integration/1(in), Trapezoid Integration/1(in)
  Merge/1 -> Rate Transition/1
  Rate Transition/1 -> Sum/1, Delay One Step/1
  Sum/1 -> sc_inc_ang_bod/1
  Delay One Step/1 -> Sum/2

== system simulator/Plant/Forces & Moments/Aerodynamics/Aerodynamic Coefficients ==
  M : Inport
  AoA : Inport  Port=2
  AoS : Inport  Port=3
  delta_ae : Inport  Port=4
  AoA Table : PreLookup  BreakpointsData=simdb.aero.AoA_table  OutputSelection=Index and fraction as bus  BeginIndexSearchUsingPreviousIndexResult=on  ExtrapMethod=Linear  RemoveProtectionInput=on
  Bus Creator : BusCreator  Inputs=8
  Demux : Demux  Outputs=5
  Drag Coefficient : Subsystem
  Lift Coefficient : Subsystem
  M Table : PreLookup  BreakpointsData=simdb.aero.M_table  OutputSelection=Index and fraction as bus  BeginIndexSearchUsingPreviousIndexResult=on  ExtrapMethod=Linear  RemoveProtectionInput=on
  Pitch Moment Coefficient : Subsystem
  Radians to Degrees : simulink_extras/Transformations/Radians to Degrees
  Radians to Degrees1 : simulink_extras/Transformations/Radians to Degrees
  Roll Moment Coefficient : Subsystem
  Sideforce Coefficient : Subsystem
  Yaw Moment Coefficient : Subsystem
  delta_b Table : PreLookup  BreakpointsData=simdb.aero.delta_b_table  OutputSelection=Index and fraction as bus  BeginIndexSearchUsingPreviousIndexResult=on  ExtrapMethod=Linear  RemoveProtectionInput=on
  delta_el Table : PreLookup  BreakpointsData=simdb.aero.delta_el_table  OutputSelection=Index and fraction as bus  BeginIndexSearchUsingPreviousIndexResult=on  ExtrapMethod=Linear  RemoveProtectionInput=on
  delta_er Table : PreLookup  BreakpointsData=simdb.aero.delta_el_table  OutputSelection=Index and fraction as bus  BeginIndexSearchUsingPreviousIndexResult=on  ExtrapMethod=Linear  RemoveProtectionInput=on
  delta_rl Table : PreLookup  BreakpointsData=simdb.aero.delta_rl_table  OutputSelection=Index and fraction as bus  BeginIndexSearchUsingPreviousIndexResult=on  ExtrapMethod=Linear  RemoveProtectionInput=on
  delta_rr Table : PreLookup  BreakpointsData=simdb.aero.delta_rl_table  OutputSelection=Index and fraction as bus  BeginIndexSearchUsingPreviousIndexResult=on  ExtrapMethod=Linear  RemoveProtectionInput=on
  CD : Outport
  CS : Outport  Port=2
  CL : Outport  Port=3
  Cl : Outport  Port=4
  Cm : Outport  Port=5
  Cn : Outport  Port=6
  wires:
  Yaw Moment Coefficient/1(Cn) -> Cn/1
  Drag Coefficient/1(CD) -> CD/1
  Pitch Moment Coefficient/1(Cm) -> Cm/1
  delta_ae/1 -> Demux/1
  AoS/1 -> Radians to Degrees1/1
  AoA/1 -> Radians to Degrees/1
  M Table/1 -> Bus Creator/1  "M"
  AoA Table/1 -> Bus Creator/2  "AoA"
  delta_el Table/1 -> Bus Creator/4  "delta_el"
  delta_er Table/1 -> Bus Creator/5  "delta_er"
  delta_rl Table/1 -> Bus Creator/6  "delta_rl"
  delta_rr Table/1 -> Bus Creator/7  "delta_rr"
  delta_b Table/1 -> Bus Creator/8  "delta_b"
  M/1 -> M Table/1
  Radians to Degrees/1 -> AoA Table/1
  Radians to Degrees1/1 -> Bus Creator/3  "AoS"
  Demux/2 -> delta_er Table/1  "delta_er"
  Demux/3 -> delta_rl Table/1  "delta_rl"
  Demux/4 -> delta_rr Table/1  "delta_rr"
  Demux/5 -> delta_b Table/1  "delta_b"
  Demux/1 -> delta_el Table/1  "delta_el"
  Lift Coefficient/1(CL) -> CL/1
  Sideforce Coefficient/1(CS) -> CS/1
  Roll Moment Coefficient/1(Cl) -> Cl/1
  Bus Creator/1 -> Yaw Moment Coefficient/1(params), Pitch Moment Coefficient/1(params), Roll Moment Coefficient/1(params), Lift Coefficient/1(params), Sideforce Coefficient/1(params), Drag Coefficient/1(params)

== system simulator/Navigation System/IMU/Accelerometer/Velocity Increment/Perfect Integration ==
  in : Inport
  Action Port : ActionPort  ActionPortLabel=case [ 2 ]:
  Integrator : Integrator
  out : Outport
  wires:
  Integrator/1 -> out/1
  in/1 -> Integrator/1

== system simulator/Navigation System/IMU/Accelerometer/Velocity Increment/Trapezoid Integration ==
  in : Inport
  Action Port : ActionPort  ActionPortLabel=case [ 1 ]:
  Delay1 : Delay  DelayLength=1
  Delay3 : Delay  DelayLength=1
  Gain : Gain  Gain=acc.internal_tsample/2
  Sum1 : Sum  Inputs=|++
  Sum3 : Sum  Inputs=|++
  out : Outport
  wires:
  Delay3/1 -> Sum3/2
  Gain/1 -> Sum3/1
  Sum1/1 -> Gain/1
  in/1 -> Sum1/2, Delay1/1
  Delay1/1 -> Sum1/1
  Sum3/1 -> out/1, Delay3/1

== system simulator/Navigation System/IMU/Gyroscope/Incremental Angle/Perfect Integration ==
  in : Inport
  Action Port : ActionPort  ActionPortLabel=case [ 2 ]:
  Integrator : Integrator
  out : Outport
  wires:
  Integrator/1 -> out/1
  in/1 -> Integrator/1

== system simulator/Navigation System/IMU/Gyroscope/Incremental Angle/Trapezoid Integration ==
  in : Inport
  Action Port : ActionPort  ActionPortLabel=case [ 1 ]:
  Delay1 : Delay  DelayLength=1
  Delay3 : Delay  DelayLength=1
  Gain : Gain  Gain=gyr.internal_tsample/2
  Sum1 : Sum  Inputs=|++
  Sum3 : Sum  Inputs=|++
  out : Outport
  wires:
  Delay3/1 -> Sum3/2
  Gain/1 -> Sum3/1
  Sum1/1 -> Gain/1
  in/1 -> Sum1/2, Delay1/1
  Delay1/1 -> Sum1/1
  Sum3/1 -> out/1, Delay3/1

== system simulator/Plant/Forces & Moments/Aerodynamics/Aerodynamic Coefficients/Drag Coefficient ==
  In Bus Element : Inport  PortName=params  Element=M
  In Bus Element1 : Inport  PortName=params  Element=AoA
  In Bus Element2 : Inport  PortName=params  Element=delta_el
  In Bus Element3 : Inport  PortName=params  Element=delta_er
  In Bus Element4 : Inport  PortName=params  Element=delta_rl
  In Bus Element5 : Inport  PortName=params  Element=delta_b
  In Bus Element6 : Inport  PortName=params  Element=delta_rr
  Add : Sum  Inputs=+++++++
  CD0 : Interpolation_n-D  Table=simdb.aero.CD0  RequireIndexFractionAsBus=on  RemoveProtectionIndex=on  InternalRulePriority=Speed
      settings: InputPortMap=u0,u1
  CDb : Interpolation_n-D  NumberOfTableDimensions=3  Table=simdb.aero.CDb  RequireIndexFractionAsBus=on  RemoveProtectionIndex=on  InternalRulePriority=Speed
      settings: InputPortMap=u0,u1,u2
  CDel : Interpolation_n-D  NumberOfTableDimensions=3  Table=simdb.aero.CDel  RequireIndexFractionAsBus=on  RemoveProtectionIndex=on  InternalRulePriority=Speed
      settings: InputPortMap=u0,u1,u2
  CDer : Interpolation_n-D  NumberOfTableDimensions=3  Table=simdb.aero.CDel  RequireIndexFractionAsBus=on  RemoveProtectionIndex=on  InternalRulePriority=Speed
      settings: InputPortMap=u0,u1,u2
  CDh : Interpolation_n-D  Commented=on  Table=simdb.aero.CDh  RequireIndexFractionAsBus=on  RemoveProtectionIndex=on  InternalRulePriority=Speed
      settings: InputPortMap=u0,u1
  CDrl : Interpolation_n-D  NumberOfTableDimensions=3  Table=simdb.aero.CDrl  RequireIndexFractionAsBus=on  RemoveProtectionIndex=on  InternalRulePriority=Speed
      settings: InputPortMap=u0,u1,u2
  CDrr : Interpolation_n-D  NumberOfTableDimensions=3  Table=simdb.aero.CDrl  RequireIndexFractionAsBus=on  RemoveProtectionIndex=on  InternalRulePriority=Speed
      settings: InputPortMap=u0,u1,u2
  Constant : Constant  Value=0
  CD : Outport
  wires:
  Add/1 -> CD/1
  Constant/1 -> Add/2
  In Bus Element/1 -> CDb/3, CDrr/3, CDrl/3, CDer/3, CDel/3, CD0/2
  In Bus Element1/1 -> CDb/1, CDrr/1, CDrl/1, CDer/1, CDel/1, CD0/1
  In Bus Element3/1 -> CDer/2
  In Bus Element2/1 -> CDel/2
  In Bus Element6/1 -> CDrr/2
  In Bus Element4/1 -> CDrl/2
  In Bus Element5/1 -> CDb/2
  CDer/1 -> Add/4
  CDel/1 -> Add/3
  CD0/1 -> Add/1
  CDrl/1 -> Add/5
  CDrr/1 -> Add/6
  CDb/1 -> Add/7

== system simulator/Plant/Forces & Moments/Aerodynamics/Aerodynamic Coefficients/Lift Coefficient ==
  In Bus Element : Inport  PortName=params  Element=M
  In Bus Element1 : Inport  PortName=params  Element=AoA
  In Bus Element2 : Inport  PortName=params  Element=delta_el
  In Bus Element3 : Inport  PortName=params  Element=delta_er
  In Bus Element4 : Inport  PortName=params  Element=delta_b
  Add1 : Sum  Inputs=++++
  CL0 : Interpolation_n-D  Table=simdb.aero.CL0  RequireIndexFractionAsBus=on  RemoveProtectionIndex=on  InternalRulePriority=Speed
      settings: InputPortMap=u0,u1
  CLb : Interpolation_n-D  NumberOfTableDimensions=3  Table=simdb.aero.CLb  RequireIndexFractionAsBus=on  RemoveProtectionIndex=on  InternalRulePriority=Speed
      settings: InputPortMap=u0,u1,u2
  CLel : Interpolation_n-D  NumberOfTableDimensions=3  Table=simdb.aero.CLel  RequireIndexFractionAsBus=on  RemoveProtectionIndex=on  InternalRulePriority=Speed
      settings: InputPortMap=u0,u1,u2
  CLer : Interpolation_n-D  NumberOfTableDimensions=3  Table=simdb.aero.CLel  RequireIndexFractionAsBus=on  RemoveProtectionIndex=on  InternalRulePriority=Speed
      settings: InputPortMap=u0,u1,u2
  CL : Outport
  wires:
  In Bus Element1/1 -> CL0/1, CLel/1, CLer/1, CLb/1
  In Bus Element/1 -> CL0/2, CLel/3, CLer/3, CLb/3
  In Bus Element4/1 -> CLb/2
  In Bus Element3/1 -> CLer/2
  In Bus Element2/1 -> CLel/2
  CLel/1 -> Add1/2
  CL0/1 -> Add1/1
  CLer/1 -> Add1/3
  CLb/1 -> Add1/4
  Add1/1 -> CL/1

== system simulator/Plant/Forces & Moments/Aerodynamics/Aerodynamic Coefficients/Pitch Moment Coefficient ==
  In Bus Element : Inport  PortName=params  Element=M
  In Bus Element1 : Inport  PortName=params  Element=AoA
  In Bus Element2 : Inport  PortName=params  Element=delta_el
  In Bus Element3 : Inport  PortName=params  Element=delta_er
  In Bus Element4 : Inport  PortName=params  Element=delta_b
  Add : Sum  Inputs=++++
  Cm0 : Interpolation_n-D  Table=simdb.aero.Cm0  RequireIndexFractionAsBus=on  RemoveProtectionIndex=on  InternalRulePriority=Speed
      settings: InputPortMap=u0,u1
  Cmb : Interpolation_n-D  NumberOfTableDimensions=3  Table=simdb.aero.Cmb  RequireIndexFractionAsBus=on  RemoveProtectionIndex=on  InternalRulePriority=Speed
      settings: InputPortMap=u0,u1,u2
  Cmel : Interpolation_n-D  NumberOfTableDimensions=3  Table=simdb.aero.Cmel  RequireIndexFractionAsBus=on  RemoveProtectionIndex=on  InternalRulePriority=Speed
      settings: InputPortMap=u0,u1,u2
  Cmer : Interpolation_n-D  NumberOfTableDimensions=3  Table=simdb.aero.Cmel  RequireIndexFractionAsBus=on  RemoveProtectionIndex=on  InternalRulePriority=Speed
      settings: InputPortMap=u0,u1,u2
  Cm : Outport
  wires:
  Add/1 -> Cm/1
  In Bus Element/1 -> Cmel/3, Cmb/3, Cmer/3, Cm0/2
  In Bus Element4/1 -> Cmb/2
  In Bus Element3/1 -> Cmer/2
  In Bus Element2/1 -> Cmel/2
  In Bus Element1/1 -> Cmb/1, Cmer/1, Cmel/1, Cm0/1
  Cmel/1 -> Add/2
  Cmer/1 -> Add/3
  Cmb/1 -> Add/4
  Cm0/1 -> Add/1

== system simulator/Plant/Forces & Moments/Aerodynamics/Aerodynamic Coefficients/Roll Moment Coefficient ==
  In Bus Element : Inport  PortName=params  Element=M
  In Bus Element1 : Inport  PortName=params  Element=AoA
  In Bus Element2 : Inport  PortName=params  Element=delta_el
  In Bus Element3 : Inport  PortName=params  Element=delta_er
  In Bus Element5 : Inport  PortName=params  Element=AoS
  Add2 : Sum  Inputs=++-
  Clb0 : Interpolation_n-D  Table=simdb.aero.Clb0  RequireIndexFractionAsBus=on  RemoveProtectionIndex=on  InternalRulePriority=Speed
      settings: InputPortMap=u0,u1
  Clel : Interpolation_n-D  NumberOfTableDimensions=3  Table=simdb.aero.Clel  RequireIndexFractionAsBus=on  RemoveProtectionIndex=on  InternalRulePriority=Speed
      settings: InputPortMap=u0,u1,u2
  Cler : Interpolation_n-D  NumberOfTableDimensions=3  Table=simdb.aero.Clel  RequireIndexFractionAsBus=on  RemoveProtectionIndex=on  InternalRulePriority=Speed
      settings: InputPortMap=u0,u1,u2
  Product : Product
  Cl : Outport
  wires:
  In Bus Element1/1 -> Cler/1, Clel/1, Clb0/1
  In Bus Element/1 -> Cler/3, Clel/3, Clb0/2
  In Bus Element3/1 -> Cler/2
  In Bus Element2/1 -> Clel/2
  Clb0/1 -> Product/2
  In Bus Element5/1 -> Product/1
  Clel/1 -> Add2/2
  Product/1 -> Add2/1
  Cler/1 -> Add2/3
  Add2/1 -> Cl/1
